simulink model "VFlexP"  (R2024a)
settings: Solver=ode23tb  StartTime=0.0  StopTime=3  FixedStep=1e-5
model workspace (MAT data in the model file):
  DCop_DCBUCK : object (value not decoded)
  Grid_CCVSC_idx = [2; 3; 4; 5; 6; 7; 8; 9; 10; 11; 12]
  Grid_CCVSCs = 1
  Grid_CCVSCs_buses = 1
  Grid_CCVSCs_toM = [0 1 0 0 0 0 0 0 0 0 0 0 ... (781 elements, 71x11)]
  Grid_C_Lines = [0 0]
  Grid_Cbuses = [0.00666666666667 0.00666666666667 0.00666666666667]
  Grid_DC : object (value not decoded)
  Grid_DCop_DCBUCK : object (value not decoded)
  Grid_DCop_DC_PES : object (value not decoded)
  Grid_DFIGs = 1
  Grid_DFIGs_buses = 1
  Grid_DGs : string (value not decoded)
  Grid_From_buses = [1 2]
  Grid_GFls = 1
  Grid_GFls_buses = 1
  Grid_GFr_idx = 1
  Grid_GFrs = 1
  Grid_GFrs_buses = 1
  Grid_GFrs_toM = [1; 0; 0]
  Grid_IG_idx = 2
  Grid_IGs = 1
  Grid_IGs_buses = 1
  Grid_IGs_toM = [0; 1]
  Grid_L_Lines = [0.05 0.05]
  Grid_L_Loads = 0
  Grid_Lines_fromM : object (value not decoded)
  Grid_Lines_toM : object (value not decoded)
  Grid_Load_buses = []
  Grid_Load_busesDC = []
  Grid_MSGs = 1
  Grid_MSGs_buses = 1
  Grid_Nbuses = 3
  Grid_PQ_gen = 3
  Grid_Ploads = []
  Grid_PloadsDC = []
  Grid_Ps_lf = -0.138475313333
  Grid_Qloads = []
  Grid_Qs_lf = 0.00594619333333
  Grid_R_Lines = [0.005 0.005]
  Grid_R_Loads = 0
  Grid_R_Loads_DC = 0
  Grid_Rcf = [150 150 150]
  Grid_SCs = 1
  Grid_SCs_buses = 1
  Grid_SG_idx = 1
  Grid_SGs = 1
  Grid_SGs_buses = 1
  Grid_SGs_toM = [1; 0]
  Grid_To_buses = [2 3]
  Grid_VCVSC_idx = [1; 2; 3; 4; 5; 6; 7; 8; 9; 10; 11; 12]
  Grid_VCVSCs = 1
  Grid_VCVSCs_buses = [1; 2; 3; 6; 8; 9; 12; 58; 59; 60; 63; 65]
  Grid_VCVSCs_toM = [1 0 0 0 0 0 0 0 0 0 0 0 ... (852 elements, 71x12)]
  Grid_VSM_idx = 2
  Grid_VSMs = 1
  Grid_VSMs_buses = 1
  Grid_VSMs_toM = [0; 1]
  Grid_admitt_matrix = [1.9801990198-19.801979198i  -1.9801980198+19.801980198i; -1.9801980198+19.801980198i  1.9801990198-19.801979198i]
  Grid_admitt_matrix_noloads = [1.9801990198-19.801979198i  -1.9801980198+19.801980198i; -1.9801980198+19.801980198i  1.9801990198-19.801979198i]
  Grid_bus = [1; 2; 3]
  Grid_busDC_complexity = 1
  Grid_busDC_complexity_PF = 2
  Grid_bus_complexity = [1 1 1]
  Grid_bus_complexity_PF = [1 1 1]
  Grid_buses_lf = 1
  Grid_conductance_matrix = 0.00666666666667
  Grid_conductance_matrix_noloads = 0.00666666666667
  Grid_fref : object (value not decoded)
  Grid_gen_static_params : mBase (value not decoded)
  Grid_iPs_lf = -7.22150378958
  Grid_iQs_lf = 168.17482109
  Grid_iadmitt_matrix = [250000.001075-249999.987531i  249999.998575-250000.012531i; 249999.998575-250000.012531i  250000.001075-249999.987531i]
  Grid_iadmitt_matrix_noloads = [250000.001075-249999.987531i  249999.998575-250000.012531i; 249999.998575-250000.012531i  250000.001075-249999.987531i]
  Grid_iconductance_matrix = 150
  Grid_iconductance_matrix_noloads = 150
  Grid_init_OK_bool = 1
  Grid_intconv_PF : object (value not decoded)
  Grid_lf_op : op_report (value not decoded)
  Grid_lineDC_complexity = []
  Grid_lineDC_complexity_PF = []
  Grid_line_complexity = [1 1]
  Grid_line_complexity_PF = [3 3]
  Grid_loadDC_complexity = []
  Grid_loadDC_complexity_PF = []
  Grid_load_complexity = []
  Grid_load_complexity_PF = []
  Grid_opDC_CCVSC : object (value not decoded)
  Grid_opDC_VSM : object (value not decoded)
  Grid_opGFr : object (value not decoded)
  Grid_opVCVSC : object (value not decoded)
  Grid_op_CCVSC : object (value not decoded)
  Grid_op_IG : object (value not decoded)
  Grid_op_SG : object (value not decoded)
  Grid_op_VSM : object (value not decoded)
  Grid_shift_lines = [0 0]
  Grid_tap_lines = [1 1]
  Grid_v_buses_mod = [1 1.0001218564 1]
  LinsysParamChangeStruct : Param1 (value not decoded)
  Lline = 0.01
  Rline = 1e-05
  linsys : object (value not decoded)
symbols that are objects in the model workspace (value not decoded): Grid_DCop_DC_PES, Grid_DCop_DCBUCK, Grid_op_CCVSC, Grid_op_IG, Grid_op_SG, Grid_op_VSM, Grid_opDC_CCVSC, Grid_opDC_VSM, Grid_opGFr, Grid_opVCVSC
undefined symbols (not defined in the file or in its folder): block_buses_DC, block_idx, CCVSC_idx, Cf, costs, costs2, DFIGs_nodes, DiscIntNeverNeededParam, entity, Fb, Fi, From_nodes, Grid_op_DFIG, Grid_op_DFIG_PQ, Grid_op_MSG, Grid_op_SC, Grid_op_VCVSC, Kic, Kiv, Kpc, Kpv, last_send, Lc, Lf, m, Matrix_flux_to_i, mD, mp, MSGs_buses, Nbuses_DC, nq, op_VCVSC, Psche, Rc, Rf, rkq1, rkq2, SCs_buses, SCs_nodes, sec_control_structure, set_DG_up, set_extra_satur, set_sending_cost, SGs_buses, SGs_nodes, Tf, To_nodes, VI_L, VI_R, WOF_Tf, xkq1, xkq2
libraries: simulink x447, eeGeneralControl x5
(part 6 of 30)

== system VFlexP/Grid/Dynamic/Generators_DC/DC_PES ==
  v : Inport
  ref : Inport  Port=2
  Gain : Gain  Gain=10
  Gain1 : Gain
  Gain4 : Gain  Gain=10
  Integrator : Integrator  InitialCondition=Grid_DCop_DC_PES.op.States(1).x'
  Integrator1 : Integrator  InitialCondition=Grid_DCop_DC_PES.op.States(2).x'
  One : Constant  Value=DC.v(block_buses)  OutDataTypeStr=Inherit: Inherit via back propagation
  Selector : Selector  InputPortWidth=DC.Nbuses  IndexOptions=Index vector (dialog)  Indices=block_buses  OutputSizes=1
  Selector1 : Selector  Commented=on  InputPortWidth=3  IndexOptions=Index vector (dialog)  Indices=[1 3]  OutputSizes=1
  State-Space : StateSpace  A=[]  B=[]  C=[]  D=block_toM  InitialCondition=0  ParameterTunability=Optimized
  Sum : Sum  Inputs=|++
  Sum1 : Sum  Inputs=|+-
  Sum3 : Sum  Inputs=|+-
  Transpose : Math  Operator=transpose
  Transpose1 : Math  Operator=transpose
  i : Outport
  wires:
  State-Space/1 -> Transpose1/1
  Transpose/1 -> State-Space/1
  Gain4/1 -> Integrator/1
  Transpose1/1 -> i/1
  Sum3/1 -> Gain1/1, Gain4/1
  ref/1 -> Selector1/1
  v/1 -> Selector/1
  Selector/1 -> Sum3/2
  One/1 -> Sum3/1
  Gain1/1 -> Sum/1
  Integrator/1 -> Sum/2
  Sum/1 -> Sum1/1
  Sum1/1 -> Gain/1
  Gain/1 -> Integrator1/1
  Integrator1/1 -> Sum1/2, Transpose/1

== system VFlexP/Grid/Dynamic/Grid/Dynamic ==
  i_from_gen : Inport
  Buses : Subsystem
  Goto Tag Visibility : GotoTagVisibility  GotoTag=Cbuses
  Lines : Subsystem
  Lines to buses : Subsystem
  Loads : Subsystem  Commented=on
  Loads to buses : Subsystem  Commented=on
  Selector2 : Selector  Commented=on  NumberOfDimensions=2  InputPortWidth=Nnodes  IndexOptions=Select all,Index vector (dialog)  Indices=1,Load_buses  OutputSizes=1,1
  Selector4 : Selector  NumberOfDimensions=2  InputPortWidth=Nnodes  IndexOptions=Select all,Index vector (dialog)  Indices=From_nodes,From_buses  OutputSizes=1,1
  Selector6 : Selector  NumberOfDimensions=2  InputPortWidth=Nnodes  IndexOptions=Select all,Index vector (dialog)  Indices=To_nodes,To_buses  OutputSizes=1,1
  Step : Step  Before=ones(1, length(From_buses))  After=[1 ones(1, length(From_buses)-1)]  SampleTime=0
  Sum : Sum  Inputs=++|
  Sum1 : Sum  Inputs=|++
  connect : Subsystem
  iCbuses : Subsystem
  iP : Subsystem  Commented=on
  v_buses : Outport
  tag scope: Cbuses=scoped
  wires:
  Buses/1(v) -> [v_buses], v_buses/1  "v"
  [i_from_lines] -> Sum/2
  [i_to_loads] -> Sum1/1
  Lines to buses/2(i_out_buses) -> [i_to_lines]
  Loads to buses/1(i_out_buses) -> [i_to_loads]
  iP/1(Out1) -> Loads/3(iP)
  Selector6/1 -> Lines/2(v_out)
  [v_buses] -> Selector2/1
  connect/1(Out1) -> Loads/2(connected)
  [v_buses] -> Selector6/1
  Loads/1(i) -> Loads to buses/1(i_loads)
  Sum/1 -> Buses/1(i_in)
  Selector4/1 -> Lines/1(v_in)
  Selector2/1 -> Loads/1(v_in)
  [v_buses] -> Selector4/1
  [i_to_lines] -> Sum1/2
  Step/1 -> iCbuses/1(In1), Lines/3(connected)
  i_from_gen/1 -> Sum/1
  Sum1/1 -> Buses/2(i_out)
  Lines to buses/1(i_in_buses) -> [i_from_lines]
  Lines/1(i) -> Lines to buses/1(i)
  iCbuses/1(Out1) -> [Cbuses]

== system VFlexP/Grid/Dynamic/Grid/Static ==
  i_from_gen : Inport
  Complex to Real-Imag : ComplexToRealImag
  Constant : Constant  Value=zeros(1, Nbuses)  VectorParams1D=off
  Gain : Gain  Gain=iadmitt_matrix  Multiplication=Matrix(K*u)
  Matrix Concatenate : Concatenate  NumInputs=3  Mode=Multidimensional array
  Real-Imag to Complex : RealImagToComplex
  Scope : Scope
  Selector : Selector  NumberOfDimensions=2  InputPortWidth=3  IndexOptions=Index vector (dialog),Select all  Indices=1,find(bus_complexity == 1)  OutputSizes=1,1
  Selector1 : Selector  NumberOfDimensions=2  InputPortWidth=3  IndexOptions=Index vector (dialog),Select all  Indices=2,find(bus_complexity == 1)  OutputSizes=1,1
  Transpose : Math  Operator=transpose
  Transpose2 : Math  Operator=transpose
  v_buses : Outport
  wires:
  Constant/1 -> Matrix Concatenate/3
  Selector/1 -> Real-Imag to Complex/1  "id1"
  Selector1/1 -> Real-Imag to Complex/2  "iq1"
  i_from_gen/1 -> Selector1/1, Selector/1
  Real-Imag to Complex/1 -> Transpose/1
  Complex to Real-Imag/1 -> Matrix Concatenate/1, Scope/1
  Complex to Real-Imag/2 -> Matrix Concatenate/2
  Transpose2/1 -> Complex to Real-Imag/1
  Transpose/1 -> Gain/1
  Gain/1 -> Transpose2/1
  Matrix Concatenate/1 -> v_buses/1

== system VFlexP/Grid/Dynamic/Grid_DC/dynamic ==
  i_from_gen_dc : Inport
  BusesDC : Subsystem
  DC_Lines_toM1 : Subsystem  TreatAsAtomicUnit=on
  DClines : Subsystem
  Loads : Subsystem  Commented=on
  Loads to buses : Subsystem  Commented=on
  One1 : Constant  Commented=on  Value=ones(1, length(R_Loads_DC))  VectorParams1D=off  OutDataTypeStr=Inherit: Inherit via back propagation
  Scope : Scope
  Selector2 : Selector  Commented=on  NumberOfDimensions=2  InputPortWidth=Nnodes  IndexOptions=Select all,Index vector (dialog)  Indices=From_nodes,DC.to  OutputSizes=1,1
  Selector4 : Selector  Commented=on  NumberOfDimensions=2  InputPortWidth=Nnodes  IndexOptions=Select all,Index vector (dialog)  Indices=From_nodes,DC.from  OutputSizes=1,1
  Selector5 : Selector  Commented=on  NumberOfDimensions=2  InputPortWidth=Nnodes  IndexOptions=Select all,Index vector (dialog)  Indices=1,Load_busesDC  OutputSizes=1,1
  Step1 : Step  Commented=on  Time=1.2  Before=zeros(1, DC.Nbuses)  After=[-0.01 zeros(1, DC.Nbuses-1)]  SampleTime=0  VectorParams1D=off
  Step3 : Step  Commented=on  Before=zeros(1, DC.Nbuses)  After=[0.01 zeros(1, DC.Nbuses-1)]  SampleTime=0  VectorParams1D=off
  Sum : Sum  Commented=on  Inputs=|++
  Sum6 : Sum  Inputs=|++
  Sum7 : Sum  Inputs=|++
  Sum8 : Sum  Inputs=|++
  v_buses_dc : Outport
  wires:
  BusesDC/1(v) -> v_buses_dc/1, [v_buses]
  [v_buses] -> Selector2/1
  Selector2/1 -> DClines/2(V_dc_out)
  Sum6/1 -> BusesDC/1(Input)
  Selector4/1 -> DClines/1(V_dc_In)
  Loads/1(i) -> Loads to buses/1(i_loads)
  Selector5/1 -> Loads/1(v_in)
  i_from_gen_dc/1 -> Sum6/2
  Sum8/1 -> BusesDC/2(Input1)
  Sum7/1 -> Sum8/1
  DC_Lines_toM1/1(i_from_lines) -> Sum6/1
  [v_buses] -> Selector4/1
  [i_to_loadsDC] -> Sum8/2
  DClines/1(i) -> DC_Lines_toM1/1(i)
  One1/1 -> Loads/2(connected)
  DC_Lines_toM1/2(i_to_lines) -> Sum7/1
  Loads to buses/1(i_out_buses) -> Scope/1, [i_to_loadsDC]
  [v_buses] -> Selector5/1
  Step3/1 -> Sum/1
  Sum/1 -> Sum7/2
  Step1/1 -> Sum/2

== system VFlexP/Grid/Dynamic/Grid_DC/static ==
  i_from_gen_dc : Inport
  Gain : Gain  Gain=iconductance_matrix  Multiplication=Matrix(K*u)
  LPF_d1 : Subsystem
  Transpose : Math  Operator=transpose
  Transpose1 : Math  Operator=transpose
  v_buses_dc : Outport
  wires:
  Gain/1 -> Transpose1/1
  LPF_d1/1(v_buses_dc) -> v_buses_dc/1
  Transpose1/1 -> LPF_d1/1(In1)
  Transpose/1 -> Gain/1
  i_from_gen_dc/1 -> Transpose/1

== system VFlexP/Grid/Dynamic/Secondary Control/MAS messages ==
  tertiary_refs : Inport
  Constant1 : Constant  Value=1000*ones(1, length(buses_lf))  VectorParams1D=off
  Constant2 : Constant  Value=100*ones(1, length(buses_lf))  VectorParams1D=off
  Costs : RandomNumber  Mean=2*ones(1,length(buses_lf))  Variance=1*ones(1,length(buses_lf))  Seed=1:length(buses_lf)  SampleTime=100  VectorParams1D=off
  Goto Tag Visibility : GotoTagVisibility  GotoTag=Pmax
  Goto Tag Visibility1 : GotoTagVisibility  GotoTag=Snom
  Goto Tag Visibility2 : GotoTagVisibility  GotoTag=costs
  ID1 : Subsystem  VariantControl=multi-agent  mask(gen_agent){ID=1, Leader=Leader, NeighN=2, Neigh1=5, Neigh2=2, Neigh3=0, Neigh4=0, Neigh5=0}
      mask prompts: ID "ID number"; Leader "Leader multi-agent"; NeighN "Number of neighbors"; Neigh1 "Neighbor 1"; Neigh2 "Neighbor 2"; Neigh3 "Neighbor 3"; Neigh4 "Neighbor 4"; Neigh5 "Neighbor 5"
      mask init:
      | block = gcb;
      | NeighN_value = str2double(NeighN);
      | bvarname = get_param(strcat(bdroot, "/", ...
      |     string(extractBetween(gcb, [bdroot '/'], '/'))), 'bvarname');
      | set_param([block '/sentToWorkspace'], 'VariableName', ['sent_' bvarname 'ID' ID])
      | set_param([block '/followingToWorkspace'], 'VariableName', ['following_' bvarname 'ID' ID])
      | set_param([block '/sendingToWorkspace'], 'VariableName', ['sending_' bvarname 'ID' ID])
      | set_param([block '/Receive'], 'MulticastTag', ...
      |     ['ID' ID])
      | set_param([block '/ID'], 'Value', ID)
      | IDnumber = str2double(ID);
      | if strcmp(Leader, "Leader")
      |     set_param([block '/Leader'], 'Value', '1')
      | else
      |     set_param([block '/Leader'], 'Value', '0')
      | end
      | bl_send = find_system(gcb, 'MatchFilter', @Simulink.match.allVariants, 'LookUnderMasks', 'on','MaskType','Send_to_neighbor');
      | 
      | set_param([block '/neigh_left'], 'Value', NeighN)
      | switch NeighN_value % Neighbors
      |     case 1
      |         for i=1:length(bl_send)
      |             set_param(bl_send{i}, 'LabelModeActiveChoice', 'one')
      |             set_param([bl_send{i} '/one/select/Neighbor'], 'const', Neigh1)
      |             set_param([bl_send{i} '/one/Cast'], 'MulticastTag', ['ID' Neigh1])
      |             set_param([bl_send{i} '/one/Castall'], 'MulticastTag', ['ID' Neigh1])
      |         end
      |     case 2
      |         for i=1:length(bl_send)
      |             set_param(bl_send{i}, 'LabelModeActiveChoice', 'two')
      |             set_param([bl_send{i} '/two/select/Neighbor1'], 'const', Neigh1)
      |             set_param([bl_send{i} '/two/Cast1'], 'MulticastTag', ['ID' Neigh1])
      |             set_param([bl_send{i} '/two/Cast1all'], 'MulticastTag', ['ID' Neigh1])
      |             set_param([bl_send{i} '/two/select/Neighbor2'], 'const', Neigh2)
      |             set_param([bl_send{i} '/two/Cast2'], 'MulticastTag', ['ID' Neigh2])
      |             set_param([bl_send{i} '/two/Cast2all'], 'MulticastTag', ['ID' Neigh2])
      |         end
      |     case 3
      |         for i=1:length(bl_send)
      |             set_param(bl_send{i}, 'LabelModeActiveChoice', 'three')
      |             set_param([bl_send{i} '/three/select/Neighbor1'], 'const', Neigh1)
      |             set_param([bl_send{i} '/three/Cast1'], 'MulticastTag', ['ID' Neigh1])
      |             set_param([bl_send{i} '/three/Cast1all'], 'MulticastTag', ['ID' Neigh1])
      |             set_param([bl_send{i} '/three/select/Neighbor2'], 'const', Neigh2)
      |             set_param([bl_send{i} '/three/Cast2'], 'MulticastTag', ['ID' Neigh2])
      |             set_param([bl_send{i} '/three/Cast2all'], 'MulticastTag', ['ID' Neigh2])
      |             set_param([bl_send{i} '/three/select/Neighbor3'], 'const', Neigh3)
      |             set_param([bl_send{i} '/three/Cast3'], 'MulticastTag', ['ID' Neigh3])
      |             set_param([bl_send{i} '/three/Cast3all'], 'MulticastTag', ['ID' Neigh3])
      |         end
      |     case 4
      |         for i=1:length(bl_send)
      |             set_param(bl_send{i}, 'LabelModeActiveChoice', 'four')
      |             set_param([bl_send{i} '/four/select/Neighbor1'], 'const', Neigh1)
      |             set_param([bl_send{i} '/four/Cast1'], 'MulticastTag', ['ID' Neigh1])
      |             set_param([bl_send{i} '/four/Cast1all'], 'MulticastTag', ['ID' Neigh1])
      |             set_param([bl_send{i} '/four/select/Neighbor2'], 'const', Neigh2)
      |             set_param([bl_send{i} '/four/Cast2'], 'MulticastTag', ['ID' Neigh2])
      |             set_param([bl_send{i} '/four/Cast2all'], 'MulticastTag', ['ID' Neigh2])
      |             set_param([bl_send{i} '/four/select/Neighbor3'], 'const', Neigh3)
      |             set_param([bl_send{i} '/four/Cast3'], 'MulticastTag', ['ID' Neigh3])
      |             set_param([bl_send{i} '/four/Cast3all'], 'MulticastTag', ['ID' Neigh3])
      |             set_param([bl_send{i} '/four/select/Neighbor4'], 'const', Neigh4)
      |             set_param([bl_send{i} '/four/Cast4'], 'MulticastTag', ['ID' Neigh4])
      |             set_param([bl_send{i} '/four/Cast4all'], 'MulticastTag', ['ID' Neigh4])
      |         end
      |     case 5
      |         for i=1:length(bl_send)
      |             set_param(bl_send{i}, 'LabelModeActiveChoice', 'five')
      |             set_param([bl_send{i} '/five/select/Neighbor1'], 'const', Neigh1)
      |             set_param([bl_send{i} '/five/Cast1'], 'MulticastTag', ['ID' Neigh1])
      |             set_param([bl_send{i} '/five/Cast1all'], 'MulticastTag', ['ID' Neigh1])
      |             set_param([bl_send{i} '/five/select/Neighbor2'], 'const', Neigh2)
      |             set_param([bl_send{i} '/five/Cast2'], 'MulticastTag', ['ID' Neigh2])
      |             set_param([bl_send{i} '/five/Cast2all'], 'MulticastTag', ['ID' Neigh2])
      |             set_param([bl_send{i} '/five/select/Neighbor3'], 'const', Neigh3)
      |             set_param([bl_send{i} '/five/Cast3'], 'MulticastTag', ['ID' Neigh3])
      |             set_param([bl_send{i} '/five/Cast3all'], 'MulticastTag', ['ID' Neigh3])
      |             set_param([bl_send{i} '/five/select/Neighbor4'], 'const', Neigh4)
      |             set_param([bl_send{i} '/five/Cast4'], 'MulticastTag', ['ID' Neigh4])
      |             set_param([bl_send{i} '/five/Cast4all'], 'MulticastTag', ['ID' Neigh4])
      |             set_param([bl_send{i} '/five/select/Neighbor5'], 'const', Neigh5)
      |             set_param([bl_send{i} '/five/Cast5'], 'MulticastTag', ['ID' Neigh5])
      |             set_param([bl_send{i} '/five/Cast5all'], 'MulticastTag', ['ID' Neigh5])
      |         end
      | end
      mask TypeOptions Leader: No leader | Leader
      mask TypeOptions NeighN: 1 | 2 | 3 | 4 | 5
      mask Callback NeighN:
      | block = gcb;
      | NeighN = str2double(get_param(block, 'NeighN'));
      | param_vis = get_param(block,'MaskVisibilities');
      | block_params = string(fieldnames(get_param(block, 'DialogParameters')));
      | param_vis(find(block_params == 'Neigh1'):find(block_params == 'Neigh5')) = cellstr("on");
      | if NeighN < 5 % Hide some
      |     param_vis(find(block_params == 'Neigh1')+NeighN:find(block_params == 'Neigh5')) = cellstr("off");
      | end
      | set_param(block,'MaskVisibilities',param_vis)
      mask DialogControl Container8 Prompt: Parameters
  ID2 : Subsystem  VariantControl=multi-agent  mask(gen_agent){ID=2, Leader=No leader, NeighN=2, Neigh1=1, Neigh2=3, Neigh3=0, Neigh4=0, Neigh5=0}
      mask prompts: ID "ID number"; Leader "Leader multi-agent"; NeighN "Number of neighbors"; Neigh1 "Neighbor 1"; Neigh2 "Neighbor 2"; Neigh3 "Neighbor 3"; Neigh4 "Neighbor 4"; Neigh5 "Neighbor 5"
      mask init: same as VFlexP/Grid/Dynamic/Secondary Control/MAS messages/ID1
      mask TypeOptions Leader: No leader | Leader
      mask TypeOptions NeighN: 1 | 2 | 3 | 4 | 5
      mask Callback NeighN:
      | block = gcb;
      | NeighN = str2double(get_param(block, 'NeighN'));
      | param_vis = get_param(block,'MaskVisibilities');
      | block_params = string(fieldnames(get_param(block, 'DialogParameters')));
      | param_vis(find(block_params == 'Neigh1'):find(block_params == 'Neigh5')) = cellstr("on");
      | if NeighN < 5 % Hide some
      |     param_vis(find(block_params == 'Neigh1')+NeighN:find(block_params == 'Neigh5')) = cellstr("off");
      | end
      | set_param(block,'MaskVisibilities',param_vis)
      mask DialogControl Container8 Prompt: Parameters
  ID3 : Subsystem  VariantControl=multi-agent  mask(gen_agent){ID=3, Leader=No leader, NeighN=2, Neigh1=2, Neigh2=4, Neigh3=0, Neigh4=0, Neigh5=0}
      mask prompts: ID "ID number"; Leader "Leader multi-agent"; NeighN "Number of neighbors"; Neigh1 "Neighbor 1"; Neigh2 "Neighbor 2"; Neigh3 "Neighbor 3"; Neigh4 "Neighbor 4"; Neigh5 "Neighbor 5"
      mask init: same as VFlexP/Grid/Dynamic/Secondary Control/MAS messages/ID1
      mask TypeOptions Leader: No leader | Leader
      mask TypeOptions NeighN: 1 | 2 | 3 | 4 | 5
      mask Callback NeighN:
      | block = gcb;
      | NeighN = str2double(get_param(block, 'NeighN'));
      | param_vis = get_param(block,'MaskVisibilities');
      | block_params = string(fieldnames(get_param(block, 'DialogParameters')));
      | param_vis(find(block_params == 'Neigh1'):find(block_params == 'Neigh5')) = cellstr("on");
      | if NeighN < 5 % Hide some
      |     param_vis(find(block_params == 'Neigh1')+NeighN:find(block_params == 'Neigh5')) = cellstr("off");
      | end
      | set_param(block,'MaskVisibilities',param_vis)
      mask DialogControl Container8 Prompt: Parameters
  ID4 : Subsystem  VariantControl=multi-agent  mask(gen_agent){ID=4, Leader=No leader, NeighN=2, Neigh1=3, Neigh2=5, Neigh3=0, Neigh4=0, Neigh5=0}
      mask prompts: ID "ID number"; Leader "Leader multi-agent"; NeighN "Number of neighbors"; Neigh1 "Neighbor 1"; Neigh2 "Neighbor 2"; Neigh3 "Neighbor 3"; Neigh4 "Neighbor 4"; Neigh5 "Neighbor 5"
      mask init: same as VFlexP/Grid/Dynamic/Secondary Control/MAS messages/ID1
      mask TypeOptions Leader: No leader | Leader
      mask TypeOptions NeighN: 1 | 2 | 3 | 4 | 5
      mask Callback NeighN:
      | block = gcb;
      | NeighN = str2double(get_param(block, 'NeighN'));
      | param_vis = get_param(block,'MaskVisibilities');
      | block_params = string(fieldnames(get_param(block, 'DialogParameters')));
      | param_vis(find(block_params == 'Neigh1'):find(block_params == 'Neigh5')) = cellstr("on");
      | if NeighN < 5 % Hide some
      |     param_vis(find(block_params == 'Neigh1')+NeighN:find(block_params == 'Neigh5')) = cellstr("off");
      | end
      | set_param(block,'MaskVisibilities',param_vis)
      mask DialogControl Container8 Prompt: Parameters
  ID5 : Subsystem  VariantControl=multi-agent  mask(gen_agent){ID=5, Leader=No leader, NeighN=2, Neigh1=4, Neigh2=1, Neigh3=0, Neigh4=0, Neigh5=0}
      mask prompts: ID "ID number"; Leader "Leader multi-agent"; NeighN "Number of neighbors"; Neigh1 "Neighbor 1"; Neigh2 "Neighbor 2"; Neigh3 "Neighbor 3"; Neigh4 "Neighbor 4"; Neigh5 "Neighbor 5"
      mask init: same as VFlexP/Grid/Dynamic/Secondary Control/MAS messages/ID1
      mask TypeOptions Leader: No leader | Leader
      mask TypeOptions NeighN: 1 | 2 | 3 | 4 | 5
      mask Callback NeighN:
      | block = gcb;
      | NeighN = str2double(get_param(block, 'NeighN'));
      | param_vis = get_param(block,'MaskVisibilities');
      | block_params = string(fieldnames(get_param(block, 'DialogParameters')));
      | param_vis(find(block_params == 'Neigh1'):find(block_params == 'Neigh5')) = cellstr("on");
      | if NeighN < 5 % Hide some
      |     param_vis(find(block_params == 'Neigh1')+NeighN:find(block_params == 'Neigh5')) = cellstr("off");
      | end
      | set_param(block,'MaskVisibilities',param_vis)
      mask DialogControl Container8 Prompt: Parameters
  Scope : Scope
  Scope1 : Scope
  Scope2 : Scope  NumInputPorts=2
  Selector : Selector  NumberOfDimensions=2  InputPortWidth=3  IndexOptions=Index vector (dialog),Select all  Indices=1:6,1  OutputSizes=1,1
  Selector1 : Selector  NumberOfDimensions=2  InputPortWidth=3  IndexOptions=Index vector (dialog),Select all  Indices=7,1  OutputSizes=1,1
  Selector2 : Selector  NumberOfDimensions=2  InputPortWidth=3  IndexOptions=Index vector (dialog),Select all  Indices=8,1  OutputSizes=1,1
  Selector3 : Selector  NumberOfDimensions=2  InputPortWidth=3  IndexOptions=Index vector (dialog),Select all  Indices=2,1  OutputSizes=1,1
  Sum of Elements : Sum  Inputs=+
  Sum of Elements1 : Sum  Inputs=+
  concat : Concatenate  NumInputs=length(buses_lf)  Mode=Multidimensional array  ConcatenateDimension=2
  secondary_refs : Outport
  tag scope: Pmax=scoped, Snom=scoped, costs=scoped
  wires:
  concat/1 -> Selector2/1, Selector1/1, Selector/1
  tertiary_refs/1 -> Selector3/1, ID1/1(in), ID2/1(in), ID3/1(in), ID4/1(in), ID5/1(in)
  Constant2/1 -> [Pmax]
  Constant1/1 -> [Snom]
  ID1/1(out) -> concat/1
  Selector/1 -> secondary_refs/1
  Selector1/1 -> Sum of Elements1/1, Scope/1
  Selector2/1 -> Scope1/1
  Selector3/1 -> Sum of Elements/1
  Sum of Elements/1 -> Scope2/1
  Sum of Elements1/1 -> Scope2/2
  Costs/1 -> [costs]
  ID2/1(out) -> concat/2
  ID3/1(out) -> concat/3
  ID4/1(out) -> concat/4
  ID5/1(out) -> concat/5

== system VFlexP/Grid/Dynamic/Secondary Control/Matrices ==
  tertiary_refs : Inport
  start_SC : Inport  Port=2
  elec : Inport  Port=3
  Gain : Gain  Gain=A_f_sc  Multiplication=Matrix(K*u)
  Gain1 : Gain  Gain=g_f_sc'
  Gain10 : Gain  Gain=[sum(A_f_sc, 2)'; sum(A_P_sc, 2)'; sum(A_v_sc, 2)'; sum(A_Q_sc, 2)']
  Gain2 : Gain  Gain=A_P_sc  Multiplication=Matrix(K*u)
  Gain3 : Gain  Gain=g_P_sc'
  Gain4 : Gain  Gain=A_v_sc  Multiplication=Matrix(K*u)
  Gain5 : Gain  Gain=g_v_sc'
  Gain6 : Gain  Gain=g_Q_sc'
  Gain7 : Gain  Gain=A_Q_sc  Multiplication=Matrix(K*u)
  Gain8 : Gain  Gain=repmat([1 0.01 1 0.01]', 1, length(buses_lf))
  Gain9 : Gain  Gain=-1
  Integrator : Integrator
  Matrix Concatenate : Concatenate  NumInputs=4  Mode=Multidimensional array
  Matrix Concatenate1 : Concatenate  NumInputs=3  Mode=Multidimensional array
  Product : Product
  Scope : Scope
  Selector : Selector  NumberOfDimensions=2  InputPortWidth=3  IndexOptions=Index vector (dialog),Select all  Indices=1,1  OutputSizes=1,1
  Selector1 : Selector  NumberOfDimensions=2  InputPortWidth=3  IndexOptions=Index vector (dialog),Select all  Indices=2,1  OutputSizes=1,1
  Selector10 : Selector  NumberOfDimensions=2  InputPortWidth=3  IndexOptions=Index vector (dialog),Select all  Indices=2,1  OutputSizes=1,1
  Selector11 : Selector  NumberOfDimensions=2  InputPortWidth=3  IndexOptions=Index vector (dialog),Select all  Indices=4,1  OutputSizes=1,1
  Selector2 : Selector  NumberOfDimensions=2  InputPortWidth=3  IndexOptions=Index vector (dialog),Select all  Indices=3,1  OutputSizes=1,1
  Selector3 : Selector  NumberOfDimensions=2  InputPortWidth=3  IndexOptions=Index vector (dialog),Select all  Indices=4,1  OutputSizes=1,1
  Selector4 : Selector  NumberOfDimensions=2  InputPortWidth=3  IndexOptions=Index vector (dialog),Select all  Indices=5,1  OutputSizes=1,1
  Selector5 : Selector  NumberOfDimensions=2  InputPortWidth=3  IndexOptions=Index vector (dialog),Select all  Indices=6,1  OutputSizes=1,1
  Selector6 : Selector  NumberOfDimensions=2  InputPortWidth=3  IndexOptions=Index vector (dialog),Select all  Indices=1:4,1  OutputSizes=1,1
  Selector7 : Selector  NumberOfDimensions=2  InputPortWidth=3  IndexOptions=Index vector (dialog),Select all  Indices=1,1  OutputSizes=1,1
  Selector8 : Selector  NumberOfDimensions=2  InputPortWidth=3  IndexOptions=Index vector (dialog),Select all  Indices=3,1  OutputSizes=1,1
  Selector9 : Selector  NumberOfDimensions=2  InputPortWidth=3  IndexOptions=Index vector (dialog),Select all  Indices=1,1  OutputSizes=1,1
  Sum{,1..3,5} (5 alike) : Sum  Inputs=|++
  Sum4 : Sum  Inputs=|-+
  Sum6 : Sum  Inputs=|+-
  Switch : Switch  Criteria=u2 > Threshold  SaturateOnIntegerOverflow=off  InputSameDT=off
  Transpose{,1..11} (12 alike) : Math  Operator=transpose
  start_SC1 : InportShadow  Port=2
  secondary_refs : Outport
  wires:
  Selector3/1 -> Transpose3/1  "Q"
  Selector/1 -> Transpose/1  "f"
  Selector1/1 -> Transpose1/1  "P"
  Selector2/1 -> Transpose2/1  "v"
  Gain/1 -> Sum/1
  Sum/1 -> Transpose4/1
  Gain1/1 -> Sum/2
  Gain2/1 -> Sum1/1
  Gain3/1 -> Sum1/2
  Sum1/1 -> Transpose5/1
  Gain4/1 -> Sum2/1
  Gain5/1 -> Sum2/2
  Gain6/1 -> Sum3/2
  Sum2/1 -> Transpose6/1
  Sum3/1 -> Transpose7/1
  Gain7/1 -> Sum3/1
  Transpose/1 -> Gain/1
  Transpose1/1 -> Gain2/1
  Transpose2/1 -> Gain4/1
  Transpose3/1 -> Gain7/1
  Transpose4/1 -> Matrix Concatenate/1
  Transpose6/1 -> Matrix Concatenate/3
  Transpose7/1 -> Matrix Concatenate/4
  Selector8/1 -> Transpose10/1
  Selector4/1 -> Matrix Concatenate1/2
  start_SC/1 -> Switch/2
  Switch/1 -> secondary_refs/1
  tertiary_refs/1 -> Switch/3, Sum5/2, Selector5/1, Selector4/1, Sum4/1
  Transpose5/1 -> Matrix Concatenate/2
  elec/1 -> Sum4/2
  Selector5/1 -> Matrix Concatenate1/3
  Selector9/1 -> Transpose8/1
  Selector10/1 -> Transpose9/1
  Selector11/1 -> Transpose11/1
  Matrix Concatenate1/1 -> Sum5/1
  Sum5/1 -> Switch/1
  Transpose8/1 -> Gain1/1
  Transpose9/1 -> Gain3/1
  Transpose10/1 -> Gain5/1
  Transpose11/1 -> Gain6/1
  Sum4/1 -> Selector6/1, Gain9/1, Selector2/1, Selector3/1, Selector1/1, Selector/1
  Integrator/1 -> Matrix Concatenate1/1
  Matrix Concatenate/1 -> Sum6/1
  Selector6/1 -> Gain10/1
  Gain9/1 -> Selector11/1, Selector8/1, Selector10/1, Selector9/1
  Product/1 -> Integrator/1
  Sum6/1 -> Selector7/1, Gain8/1
  Selector7/1 -> Scope/1
  Gain8/1 -> Product/1
  start_SC1/1 -> Product/2
  Gain10/1 -> Sum6/2

== system VFlexP/Grid/Dynamic/Secondary Control/Matrices with delay ==
  tertiary_refs : Inport
  elec : Inport  Port=2
  start_SC : Inport  Port=3
  Assignment : Assignment  NumberOfDimensions=2  DiagnosticForDimensions=Warning  IndexOptions=Index vector (dialog),Assign all  Indices=1,1  OutputSizes=1,1
  Assignment1 : Assignment  NumberOfDimensions=2  DiagnosticForDimensions=Warning  IndexOptions=Index vector (dialog),Assign all  Indices=2,1  OutputSizes=1,1
  For Each Subsystem : Subsystem  TreatAsAtomicUnit=on  mask{delayM=delayM, A_f_sc=A_f_sc}
  For Each Subsystem1 : Subsystem  TreatAsAtomicUnit=on  mask{delayM=delayM, A_P_sc=A_P_sc}
  For Each Subsystem2 : Subsystem  TreatAsAtomicUnit=on  mask{delayM=delayM, A_v_sc=A_v_sc}
  For Each Subsystem3 : Subsystem  TreatAsAtomicUnit=on  mask{delayM=delayM, A_Q_sc=A_Q_sc}
  Gain : Gain  Gain=-1
  Gain1 : Gain  Gain=g_f_sc'
  Gain2 : Gain  Gain=[sum(A_f_sc, 2)'; sum(A_P_sc, 2)'; sum(A_v_sc, 2)'; sum(A_Q_sc, 2)']
  Gain3 : Gain  Gain=g_P_sc'
  Gain5 : Gain  Gain=g_v_sc'
  Gain6 : Gain  Gain=g_Q_sc'
  Gain8 : Gain
  Integrator : Integrator
  Matrix Concatenate : Concatenate  NumInputs=4  Mode=Multidimensional array
  Matrix Concatenate1 : Concatenate  NumInputs=3  Mode=Multidimensional array
  Selector : Selector  NumberOfDimensions=2  InputPortWidth=3  IndexOptions=Index vector (dialog),Select all  Indices=1,1  OutputSizes=1,1
  Selector1 : Selector  NumberOfDimensions=2  InputPortWidth=3  IndexOptions=Index vector (dialog),Select all  Indices=2,1  OutputSizes=1,1
  Selector10 : Selector  NumberOfDimensions=2  InputPortWidth=3  IndexOptions=Index vector (dialog),Select all  Indices=2,1  OutputSizes=1,1
  Selector11 : Selector  NumberOfDimensions=2  InputPortWidth=3  IndexOptions=Index vector (dialog),Select all  Indices=4,1  OutputSizes=1,1
  Selector12 : Selector  NumberOfDimensions=2  InputPortWidth=3  IndexOptions=Index vector (dialog),Select all  Indices=2,1  OutputSizes=1,1
  Selector2 : Selector  NumberOfDimensions=2  InputPortWidth=3  IndexOptions=Index vector (dialog),Select all  Indices=3,1  OutputSizes=1,1
  Selector3 : Selector  NumberOfDimensions=2  InputPortWidth=3  IndexOptions=Index vector (dialog),Select all  Indices=4,1  OutputSizes=1,1
  Selector4 : Selector  NumberOfDimensions=2  InputPortWidth=3  IndexOptions=Index vector (dialog),Select all  Indices=6,1  OutputSizes=1,1
  Selector5 : Selector  NumberOfDimensions=2  InputPortWidth=3  IndexOptions=Index vector (dialog),Select all  Indices=5,1  OutputSizes=1,1
  Selector6 : Selector  NumberOfDimensions=2  InputPortWidth=3  IndexOptions=Index vector (dialog),Select all  Indices=1:4,1  OutputSizes=1,1
  Selector7 : Selector  NumberOfDimensions=2  InputPortWidth=3  IndexOptions=Index vector (dialog),Select all  Indices=1,1  OutputSizes=1,1
  Selector8 : Selector  NumberOfDimensions=2  InputPortWidth=3  IndexOptions=Index vector (dialog),Select all  Indices=3,1  OutputSizes=1,1
  Selector9 : Selector  NumberOfDimensions=2  InputPortWidth=3  IndexOptions=Index vector (dialog),Select all  Indices=1,1  OutputSizes=1,1
  Sum{,1..3,5,7..8} (7 alike) : Sum  Inputs=|++
  Sum of Elements{,1..3} (4 alike) : Sum  Inputs=+  CollapseMode=Specified dimension  CollapseDim=2
  Sum4 : Sum  Inputs=|-+
  Sum6 : Sum  Inputs=|+-
  Switch : Switch  Criteria=u2 > Threshold  SaturateOnIntegerOverflow=off  InputSameDT=off
  Transpose{,1..11} (12 alike) : Math  Operator=transpose
  Zero : Constant  Value=zeros(1, length(buses_lf))  VectorParams1D=off  OutDataTypeStr=Inherit: Inherit via back propagation
  secondary_refs : Outport
  wires:
  Selector3/1 -> Transpose3/1  "Q"
  Selector/1 -> Transpose/1  "f"
  Selector1/1 -> Transpose1/1  "P"
  Selector2/1 -> Transpose2/1  "v"
  Selector4/1 -> Matrix Concatenate1/3
  Sum/1 -> Transpose4/1
  Gain1/1 -> Sum/2
  Gain3/1 -> Sum1/2
  Sum1/1 -> Transpose5/1
  Sum of Elements2/1 -> Sum2/1
  Gain5/1 -> Sum2/2
  Gain6/1 -> Sum3/2
  Sum2/1 -> Transpose6/1
  Sum3/1 -> Transpose7/1
  Sum of Elements3/1 -> Sum3/1
  Transpose/1 -> For Each Subsystem/1(In1)
  Transpose1/1 -> For Each Subsystem1/1(In1)
  Transpose2/1 -> For Each Subsystem2/1(In1)
  Transpose3/1 -> For Each Subsystem3/1(In1)
  Transpose4/1 -> Matrix Concatenate/1
  Transpose6/1 -> Matrix Concatenate/3
  Transpose7/1 -> Matrix Concatenate/4
  For Each Subsystem/1(Out1) -> Sum of Elements/1
  For Each Subsystem1/1(Out1) -> Sum of Elements1/1
  For Each Subsystem2/1(Out1) -> Sum of Elements2/1
  For Each Subsystem3/1(Out1) -> Sum of Elements3/1
  Switch/1 -> secondary_refs/1
  Transpose5/1 -> Matrix Concatenate/2
  tertiary_refs/1 -> Sum5/2, Switch/3, Selector4/1, Selector5/1, Sum4/1
  elec/1 -> Sum4/2
  Matrix Concatenate1/1 -> Sum5/1
  Sum5/1 -> Switch/1
  Selector10/1 -> Transpose9/1
  Selector8/1 -> Transpose10/1
  Selector11/1 -> Transpose11/1
  Sum4/1 -> Gain/1, Selector2/1, Selector6/1, Selector3/1, Selector1/1, Selector/1
  Selector9/1 -> Transpose8/1
  Sum6/1 -> Gain8/1
  Matrix Concatenate/1 -> Sum6/1
  Selector6/1 -> Gain2/1
  start_SC/1 -> Switch/2
  Transpose8/1 -> Gain1/1
  Transpose9/1 -> Gain3/1
  Transpose10/1 -> Gain5/1
  Transpose11/1 -> Gain6/1
  Gain/1 -> Selector11/1, Selector8/1, Selector10/1, Selector9/1
  Integrator/1 -> Matrix Concatenate1/1
  Gain8/1 -> Integrator/1
  Selector5/1 -> Matrix Concatenate1/2
  Gain2/1 -> Selector7/1, Selector12/1, Assignment/1
  Zero/1 -> Assignment/2
  Assignment/1 -> Assignment1/1
  Selector7/1 -> Sum7/1
  Selector12/1 -> Sum7/2
  Sum7/1 -> Assignment1/2
  Assignment1/1 -> Sum6/2
  Sum of Elements/1 -> Sum8/1
  Sum8/1 -> Sum1/1
  Sum of Elements1/1 -> Sum8/2

== system VFlexP/Grid/Dynamic/Secondary Control/Matrices with delay and limitation ==
  tertiary_refs : Inport
  elec : Inport  Port=2
  start_SC : Inport  Port=3
  Abs : Abs  SaturateOnIntegerOverflow=off
  Constant : Constant  Value=ones(2, length(buses_lf))  VectorParams1D=off
  Constant1 : Constant  Value=costs'  VectorParams1D=off
  Constant16 : Constant  Value=sec_control_structure
  Constant17 : Constant  Value=costs'  VectorParams1D=off
  Constant19 : Constant  VectorParams1D=off
  Constant2 : Constant  Value=2*costs'  VectorParams1D=off
  Constant3 : Constant
  Display : Display
  Divide : Product  Inputs=*/
  For Each Subsystem : Subsystem  TreatAsAtomicUnit=on  mask{delayM=delayM, A_f_sc=A_f_sc}
  For Each Subsystem1 : Subsystem  TreatAsAtomicUnit=on  mask{delayM=delayM, A_P_sc=A_P_sc}
  For Each Subsystem2 : Subsystem  TreatAsAtomicUnit=on  mask{delayM=delayM, A_v_sc=A_v_sc}
  For Each Subsystem3 : Subsystem  TreatAsAtomicUnit=on  mask{delayM=delayM, A_Q_sc=A_Q_sc}
  Gain : Gain  Gain=-2
  Gain1 : Gain  Gain=g_f_sc'
  Gain11 : Gain  Gain=1/100
  Gain3 : Gain  Gain=g_P_sc'
  Gain4 : Gain  Gain=1/100
  Gain5 : Gain  Gain=g_v_sc'
  Gain6 : Gain  Gain=g_Q_sc'
  Gain7 : Gain  Gain=repmat([1; 1.01; 1; 1], 1, 4)
  Gain8 : Gain  Gain=repmat([0 0.1 1 0.1]', 1, length(buses_lf))
  Goto Tag Visibility : GotoTagVisibility  GotoTag=Pref
  Goto Tag Visibility1 : GotoTagVisibility  GotoTag=Qref
  Goto Tag Visibility2 : GotoTagVisibility  GotoTag=ielec
  Goto Tag Visibility3 : GotoTagVisibility  GotoTag=leader
  Integrator : Integrator
  Matrix Concatenate : Concatenate  NumInputs=4  Mode=Multidimensional array
  Matrix Concatenate1 : Concatenate  Mode=Multidimensional array
  Matrix Concatenate2 : Concatenate  Mode=Multidimensional array
  Matrix Concatenate3 : Concatenate  Mode=Multidimensional array
  Multiport Switch : MultiPortSwitch  Inputs=5  SaturateOnIntegerOverflow=off  InputSameDT=off
  One3 : Constant  OutDataTypeStr=Inherit: Inherit via back propagation
  Product : Product  Inputs=3
  Product{1..2,13..14} (4 alike) : Product
  Scope : Scope
  Selector : Selector  NumberOfDimensions=2  InputPortWidth=3  IndexOptions=Index vector (dialog),Select all  Indices=1,1  OutputSizes=1,1
  Selector{1,4,10,13,18} (5 alike) : Selector  NumberOfDimensions=2  InputPortWidth=3  IndexOptions=Index vector (dialog),Select all  Indices=2,1  OutputSizes=1,1
  Selector11 : Selector  NumberOfDimensions=2  InputPortWidth=3  IndexOptions=Index vector (dialog),Select all  Indices=4,1  OutputSizes=1,1
  Selector12 : Selector  NumberOfDimensions=2  InputPortWidth=3  IndexOptions=Index vector (dialog),Select all  Indices=5:6,1  OutputSizes=1,1
  Selector14 : Selector  NumberOfDimensions=2  InputPortWidth=3  IndexOptions=Index vector (dialog),Index vector (dialog)  Indices=2,1  OutputSizes=1,1
  Selector15 : Selector  NumberOfDimensions=2  InputPortWidth=3  IndexOptions=Index vector (dialog),Select all  Indices=1:4,1  OutputSizes=1,1
  Selector2 : Selector  NumberOfDimensions=2  InputPortWidth=3  IndexOptions=Index vector (dialog),Select all  Indices=3,1  OutputSizes=1,1
  Selector3 : Selector  NumberOfDimensions=2  InputPortWidth=3  IndexOptions=Index vector (dialog),Select all  Indices=4,1  OutputSizes=1,1
  Selector6 : Selector  NumberOfDimensions=2  InputPortWidth=3  IndexOptions=Index vector (dialog),Select all  Indices=1:4,1  OutputSizes=1,1
  Selector7 : Selector  NumberOfDimensions=2  InputPortWidth=3  IndexOptions=Index vector (dialog),Select all  Indices=4,1  OutputSizes=1,1
  Selector8 : Selector  NumberOfDimensions=2  InputPortWidth=3  IndexOptions=Index vector (dialog),Select all  Indices=3,1  OutputSizes=1,1
  Selector9 : Selector  NumberOfDimensions=2  InputPortWidth=3  IndexOptions=Index vector (dialog),Select all  Indices=1,1  OutputSizes=1,1
  Subsystem : Subsystem
  Sum{,1..3,5,7} (6 alike) : Sum  Inputs=|++
  Sum of Elements{,1..3} (4 alike) : Sum  Inputs=+  CollapseMode=Specified dimension  CollapseDim=2
  Sum4 : Sum  Inputs=|-+
  Sum6 : Sum  Inputs=|+-
  Switch : Switch  Criteria=u2 > Threshold  SaturateOnIntegerOverflow=off  InputSameDT=off
  Switch1 : Switch  Criteria=u2 > Threshold  SaturateOnIntegerOverflow=off  InputSameDT=off
  Switch2 : Switch  Criteria=u2 > Threshold  SaturateOnIntegerOverflow=off  InputSameDT=off
  Switch3 : Switch  Criteria=u2 > Threshold  Threshold=1  SaturateOnIntegerOverflow=off  InputSameDT=off
  Transport Delay : TransportDelay  DelayTime=1e-9
  Transpose{,1..11} (12 alike) : Math  Operator=transpose
  Zero : Constant  Value=zeros(2, length(buses_lf))  VectorParams1D=off  OutDataTypeStr=Inherit: Inherit via back propagation
  limitation : Subsystem
  secondary_refs : Outport
  tag scope: Pref=scoped, Qref=scoped, ielec=scoped, leader=scoped
  wires:
  Selector3/1 -> Transpose3/1  "Q"
  Selector/1 -> Transpose/1  "f"
  Product2/1 -> Transpose1/1  "P"
  Selector2/1 -> Transpose2/1  "v"
  Sum/1 -> Transpose4/1
  Gain1/1 -> Sum/2
  Sum of Elements1/1 -> Sum1/1
  Gain3/1 -> Sum1/2
  Sum1/1 -> Transpose5/1
  Sum of Elements2/1 -> Sum2/1
  Gain5/1 -> Sum2/2
  Gain6/1 -> Sum3/2
  Sum2/1 -> Transpose6/1
  Sum3/1 -> Transpose7/1
  Sum of Elements3/1 -> Sum3/1
  Transpose/1 -> For Each Subsystem/1(In1)
  Transpose1/1 -> For Each Subsystem1/1(In1)
  Transpose2/1 -> For Each Subsystem2/1(In1)
  Transpose3/1 -> For Each Subsystem3/1(In1)
  Transpose4/1 -> Matrix Concatenate/1
  Transpose6/1 -> Matrix Concatenate/3
  Transpose7/1 -> Matrix Concatenate/4
  Sum of Elements/1 -> Sum/1
  For Each Subsystem/1(Out1) -> Sum of Elements/1
  For Each Subsystem1/1(Out1) -> Sum of Elements1/1
  For Each Subsystem2/1(Out1) -> Sum of Elements2/1
  For Each Subsystem3/1(Out1) -> Sum of Elements3/1
  Switch/1 -> Selector14/1, Display/1, secondary_refs/1
  Transpose5/1 -> Matrix Concatenate/2
  Matrix Concatenate1/1 -> Sum5/1
  Sum5/1 -> Switch/1
  Selector10/1 -> Transpose9/1
  Selector8/1 -> Transpose10/1
  Selector11/1 -> Transpose11/1
  Switch1/1 -> Selector2/1, Selector3/1, Selector1/1, Selector/1
  Selector9/1 -> Transpose8/1
  Matrix Concatenate/1 -> Transport Delay/1, Sum6/1
  Selector6/1 -> Sum6/2
  start_SC/1 -> Product/3, Switch/2
  Transpose8/1 -> Gain1/1
  Transpose9/1 -> Gain3/1
  Transpose10/1 -> Gain5/1
  Transpose11/1 -> Gain6/1
  Gain/1 -> Selector11/1, Selector8/1, Selector10/1, Selector9/1
  Selector13/1 -> [Pref]
  Selector7/1 -> [Qref]
  limitation/1(Out1) -> [awup]
  limitation/2(Out2) -> Matrix Concatenate1/1
  Gain8/1 -> Product/1
  Matrix Concatenate2/1 -> Switch1/2
  [awup] -> Matrix Concatenate2/1
  Constant/1 -> Matrix Concatenate2/2
  Sum4/1 -> Switch1/1, Selector15/1, Gain/1, Selector12/1, Selector4/1, Selector6/1
  Selector12/1 -> Matrix Concatenate3/2
  Transport Delay/1 -> Gain7/1
  Selector14/1 -> Scope/1
  Subsystem/1(leader) -> [leader]
  Selector15/1 -> [ielec]
  tertiary_refs/1 -> Sum5/2, Switch/3, Selector7/1, Selector13/1, Sum4/1
  Zero/1 -> Matrix Concatenate1/2
  Sum6/1 -> Gain8/1
  Integrator/1 -> limitation/1(In1)
  Product/1 -> Integrator/1
  [awup] -> Product/2
  elec/1 -> Selector18/1, Subsystem/1(In1), Sum4/2
  Sum7/1 -> Gain11/1
  Gain4/1 -> Multiport Switch/3, Product14/2, Product14/1
  Gain11/1 -> Multiport Switch/5, Product13/2, Product13/1
  One3/1 -> Switch3/3
  Constant1/1 -> Sum7/1
  Constant16/1 -> Switch3/2, Multiport Switch/1
  [gaincost] -> Product2/2
  Selector4/1 -> Switch2/2
  Multiport Switch/1 -> Divide/2, Switch2/1
  Selector18/1 -> Abs/1
  Product1/1 -> Sum7/2
  Product13/1 -> Multiport Switch/6
  Divide/1 -> Switch3/1
  Switch3/1 -> Switch2/3
  Switch2/1 -> [gaincost]
  Constant3/1 -> Multiport Switch/2
  Product14/1 -> Multiport Switch/4
  Constant2/1 -> Product1/1
  Constant19/1 -> Divide/1
  Constant17/1 -> Gain4/1
  Selector1/1 -> Product2/1  "P"
  Matrix Concatenate3/1 -> Switch1/3
  Gain7/1 -> Matrix Concatenate3/1
  Abs/1 -> Product1/2
